simulink model "main_sim"  (R2022a)
settings: Solver=ode4  StartTime=t_inicial  StopTime=t_final  FixedStep=t_step  RelTol=1e-3
undefined symbols (not defined in the file): ai, As, bi, Bs, Cs, Ds, L, lambdai, mi, n_max, n_modos, side, tac, v0, v0p, vi, wi, x0
settings Model: VariantFading=off  Creator=LEGION  LastModifiedBy=LEGION

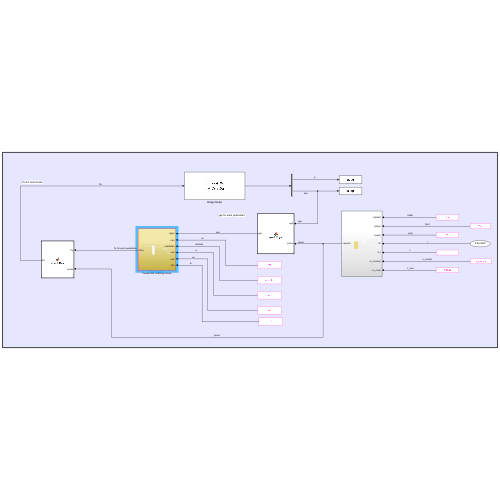
[thumbnail: Simulink's stored preview of the top-level diagram]
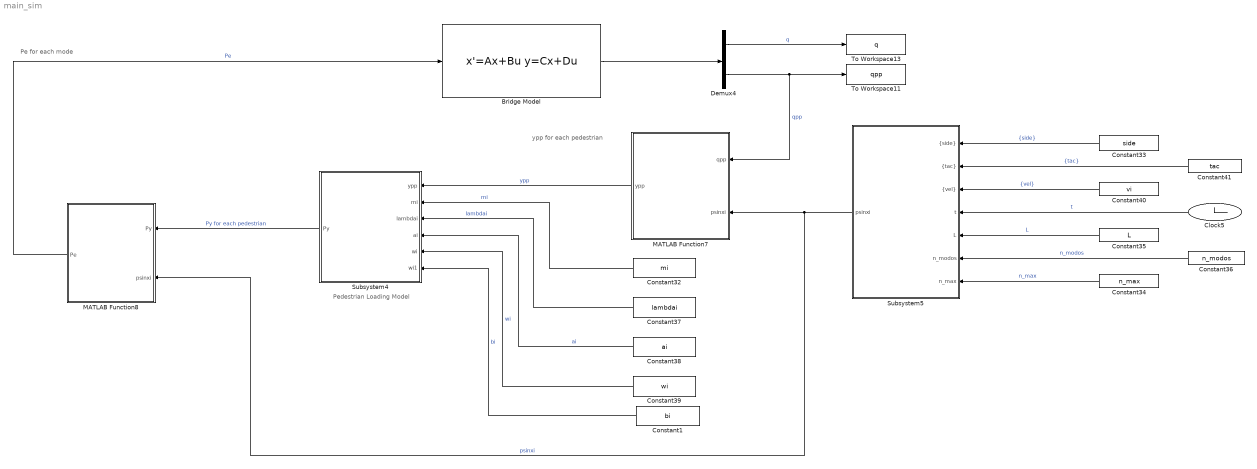
== system main_sim ==
  note: Pedestrian Loading Model
  note: Pe for each mode
  note: ypp for each pedestrian
  Bridge Model : StateSpace  A=As  B=Bs  C=Cs  D=Ds  InitialCondition=x0
  Clock5 : Clock
  Constant1 : Constant  Value=bi
  Constant32 : Constant  Value=mi
  Constant33 : Constant  Value=side
  Constant34 : Constant  Value=n_max
  Constant35 : Constant  Value=L
  Constant36 : Constant  Value=n_modos
  Constant37 : Constant  Value=lambdai
  Constant38 : Constant  Value=ai
  Constant39 : Constant  Value=wi
  Constant40 : Constant  Value=vi
  Constant41 : Constant  Value=tac
  Demux4 : Demux  Outputs=2
  MATLAB Function7 : MATLAB Function  TreatAsAtomicUnit=on
  MATLAB Function8 : MATLAB Function  TreatAsAtomicUnit=on
  Subsystem4 : Subsystem
  Subsystem5 : Subsystem
  To Workspace11 : ToWorkspace  VariableName=qpp  SaveFormat=Timeseries  SampleTime=-1
  To Workspace13 : ToWorkspace  VariableName=q  SaveFormat=Timeseries  SampleTime=-1
  wires:
  Bridge Model/1 -> Demux4/1
  MATLAB Function7/1(ypp) -> Subsystem4/1(ypp)  "ypp"
  Constant38/1 -> Subsystem4/4(ai)  "ai"
  Constant37/1 -> Subsystem4/3(lambdai)  "lambdai"
  Constant32/1 -> Subsystem4/2(mi)  "mi"
  Constant34/1 -> Subsystem5/7(n_max)  "n_max"
  Subsystem5/1(psinxi) -> MATLAB Function8/2(psinxi), MATLAB Function7/2(psinxi)  "psinxi"
  Demux4/2 -> To Workspace11/1, MATLAB Function7/1(qpp)  "qpp"
  Constant33/1 -> Subsystem5/1("{side}")  "{side}"
  Constant40/1 -> Subsystem5/3("{vel}")  "{vel}"
  Constant36/1 -> Subsystem5/6(n_modos)  "n_modos"
  Constant39/1 -> Subsystem4/5(wi)  "wi"
  Demux4/1 -> To Workspace13/1  "q"
  Constant41/1 -> Subsystem5/2("{tac}")  "{tac}"
  Subsystem4/1(Py) -> MATLAB Function8/1(Py)  "Py for each pedestrian"
  MATLAB Function8/1(Pe) -> Bridge Model/1  "Pe"
  Constant35/1 -> Subsystem5/5(L)  "L"
  Clock5/1 -> Subsystem5/4(t)  "t"
  Constant1/1 -> Subsystem4/6(wi1)  "bi"

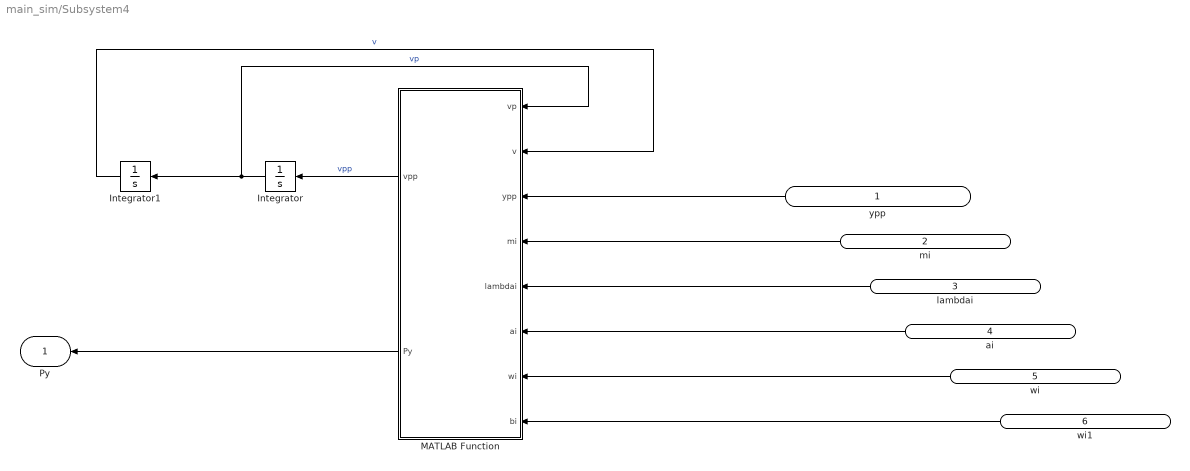
== system main_sim/Subsystem4 ==
  ypp : Inport
  mi : Inport  Port=2
  lambdai : Inport  Port=3
  ai : Inport  Port=4
  wi : Inport  Port=5
  wi1 : Inport  Port=6
  Integrator : Integrator  InitialCondition=v0p
  Integrator1 : Integrator  InitialCondition=v0
  MATLAB Function : MATLAB Function  TreatAsAtomicUnit=on
  Py : Outport
  wires:
  MATLAB Function/1(vpp) -> Integrator/1  "vpp"
  Integrator/1 -> MATLAB Function/1(vp), Integrator1/1  "vp"
  ypp/1 -> MATLAB Function/3(ypp)
  Integrator1/1 -> MATLAB Function/2(v)  "v"
  mi/1 -> MATLAB Function/4(mi)
  lambdai/1 -> MATLAB Function/5(lambdai)
  ai/1 -> MATLAB Function/6(ai)
  wi/1 -> MATLAB Function/7(wi)
  MATLAB Function/2(Py) -> Py/1
  wi1/1 -> MATLAB Function/8(bi)

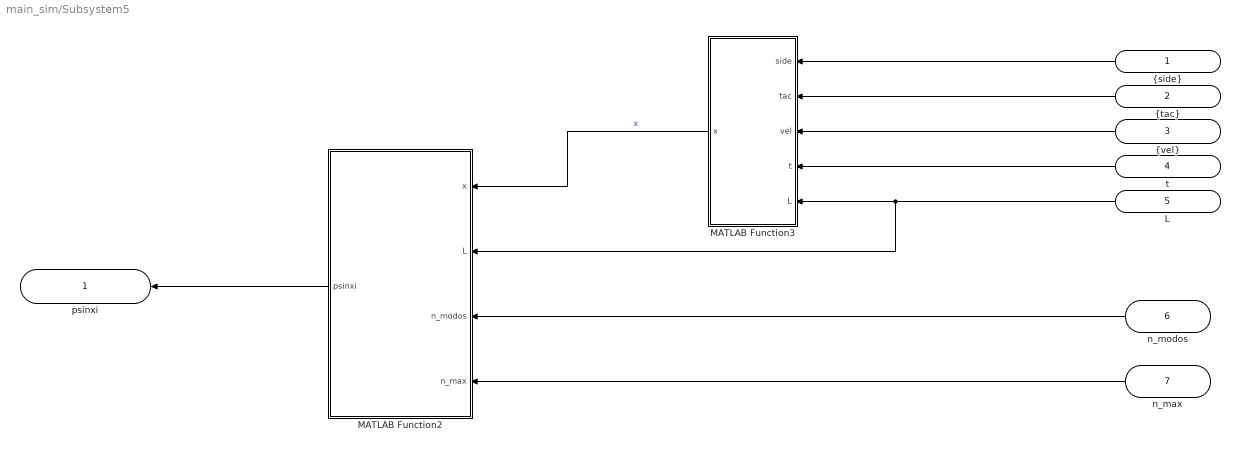
== system main_sim/Subsystem5 ==
  "{side}" : Inport
  "{tac}" : Inport  Port=2
  "{vel}" : Inport  Port=3
  t : Inport  Port=4
  L : Inport  Port=5
  n_modos : Inport  Port=6
  n_max : Inport  Port=7
  MATLAB Function2 : MATLAB Function  TreatAsAtomicUnit=on
  MATLAB Function3 : MATLAB Function  TreatAsAtomicUnit=on
  psinxi : Outport
  wires:
  L/1 -> MATLAB Function3/5(L), MATLAB Function2/2(L)
  MATLAB Function3/1(x) -> MATLAB Function2/1(x)  "x"
  n_modos/1 -> MATLAB Function2/3(n_modos)
  "{side}"/1 -> MATLAB Function3/1(side)
  MATLAB Function2/1(psinxi) -> psinxi/1
  "{tac}"/1 -> MATLAB Function3/2(tac)
  t/1 -> MATLAB Function3/4(t)
  "{vel}"/1 -> MATLAB Function3/3(vel)
  n_max/1 -> MATLAB Function2/4(n_max)

== matlab function main_sim/MATLAB Function7 ==
  data: qpp input; psinxi input; ypp output
function ypp = genToPhys(qpp,psinxi)
% Generar la aceleración que expermentan todos los peatones i (desde el 1
% hasta el peatón p), sumando la respuesta modal de todos los modos (la
% contribución modal)
% ypp = sum(psinxi*qpp,2);                                                    % Sumo todas las contribuciones modales de cada modo
ypp = psinxi*qpp;

== matlab function main_sim/MATLAB Function8 ==
  data: Py input; Pe output; psinxi input
function Pe = physToGen(Py,psinxi)
Pe = psinxi.'*Py;                                                           % Utilicé .' en vez de ' solamente ya que por experiencia me da error a veces si solo ocupo '

== matlab function main_sim/Subsystem4/MATLAB Function ==
  data: vp input; v input; ypp input; vpp output; mi input; lambdai input; ai input; wi input; Py output; bi input
function [vpp,Py] = fcn(vp,v,ypp,mi,lambdai,ai,wi,bi)

% Parámetros iniciales
% bi = 2*pi;  
A = ones(length(bi),1)./(bi.^2);                                                   % Ver modifiedVanDerPolTypeWalker.m
lambda1 = lambdai./(bi.*(A.^2));
lambda2 = lambdai.*(bi)./(A.^2);
lambda3 = lambdai.*bi;
wi = wi./(2*pi).*bi;

% Van Der Pol Type Walker Modificado
fvdv = (lambda1.*(vp.^2) + lambda2.*(v.^2) - lambda3.*ai).*vp + (wi.^2).*v;

% Aceleración del peatón
vpp = -ypp -fvdv;

% Fuerza que aplica el peatón sobre el puente
Py = -mi.*vpp;

== matlab function main_sim/Subsystem5/MATLAB Function2 ==
  data: x input; psinxi output; L input; n_modos input; n_max input
function psinxi = psinxi(x,L,n_modos,n_max)
    %% Primera forma de hacerlo
% %    psinxi = zeros(n_max,n_modos);
%     
%     % Formar matriz M
%     M = pi/L*ones(n_max,1)*(1:1:n_modos);                                       % Matriz [M]
%     
%     % Formar psinxi
%     psinxi = sin(M.*x);                                                         % [psi_n(x_i)] = sin([M]*{x})
    
    %% Tercera formaforma de hacerlo  (con esta si funciona)
    %Recorriendo cada modo
%     psinxi = zeros(n_max,n_modos);
    psinxi = zeros(200,2);                                                  %%%%%%%%%%% YA SE ME HABÍA OLVIDADO, CUIDADO CON LA CANTIDAD DE PEATONES Y LA CANTIDAD DE MODOS
    for n = 1:n_modos
        psinxi(:,n) = sin(pi*n/L*x);
    end

== matlab function main_sim/Subsystem5/MATLAB Function3 ==
  data: side input; x output; tac input; vel input; t input; L input
function x = posi(side,tac,vel,t,L)
% Determinar la posición del peatón para cada tiempo

pd = length(side);                                                          % cantidad de peatones
x0 = L*ones(pd,1).*(side-ones(pd,1));                                       % Posición inicial (izquierda o derecha)
x = zeros(pd,1);                                                            % posición
x_ = zeros(pd,1);                                                           % posición auxiliar

for i = 1:pd                                                                % Para cada peatón
    if t < tac(i)                                                           % Si aun no entra 
        delta1 = 0;
        delta2 = 0;
    else                                                                    % Si entró
        delta1 = 1;
        delta2 = t - tac(i);
    end
%     x_(i) = x0(i)*delta1 + vel(i)*delta2;
    x_(i) = x0(i)*delta1 + vel(i)*delta2;                                   % Distancia recorrida desde ese extremo (posición auxiliar
    n = floor(x_(i)/L);                                                     % Cantidad de veces que posición auxiliar superó el largo del puente
    if rem(n,2) == 0                                                        % Si es par
        x(i) = x_(i) - n*L;
    elseif rem(n,2) == 1                                                    % Si es impar
        x(i) = (n+1)*L - x_(i);
    end
end
